simulink subsystem "Voice"  (R2023b)
settings: Solver=VariableStepAuto  StartTime=0.0  StopTime=10.0  RelTol=1e-3
model mask{rng_seeds=0, sample_dim_f=0}
  mask prompts: rng_seeds "rng seeds"; sample_dim_f "sample dim"
settings Model: Creator=Edp  LastModifiedBy=giorg

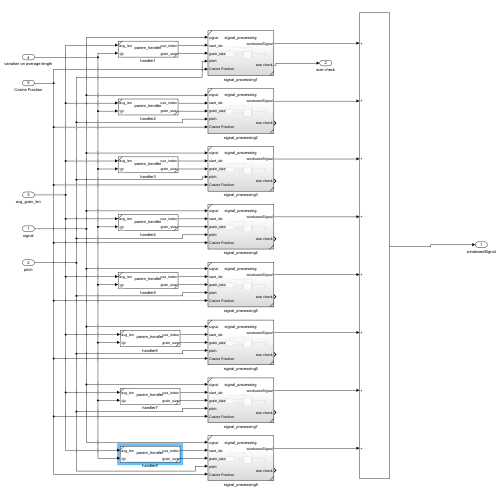
[thumbnail: Simulink's stored preview of the top-level diagram]
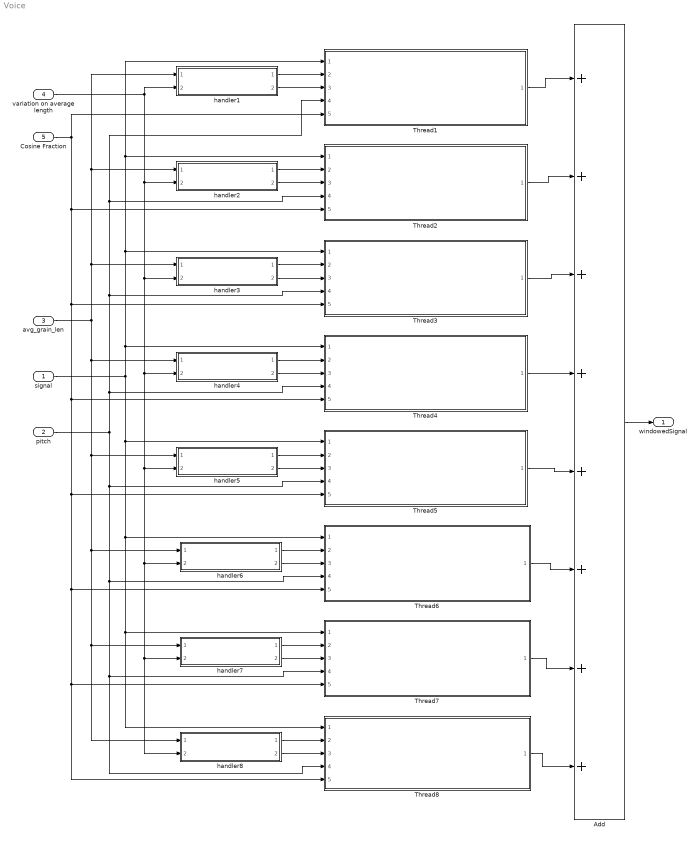
== system Voice ==
  signal : Inport
  pitch : Inport  Port=2
  avg_grain_len : Inport  Port=3
  variation on average length : Inport  Port=4
  Cosine Fraction : Inport  Port=5
  Add : Sum  Inputs=++++++++
  Thread{1..8} (8 alike) : Subsystem  ReferencedSubsystem=thread
  handler1 : Subsystem  ReferencedSubsystem=param_handler  rng_seed_f=rng_seeds(1)  sample_dim_f=sample_dim_f
  handler2 : Subsystem  ReferencedSubsystem=param_handler  rng_seed_f=rng_seeds(2)  sample_dim_f=sample_dim_f
  handler3 : Subsystem  ReferencedSubsystem=param_handler  rng_seed_f=rng_seeds(3)  sample_dim_f=sample_dim_f
  handler4 : Subsystem  ReferencedSubsystem=param_handler  rng_seed_f=rng_seeds(4)  sample_dim_f=sample_dim_f
  handler5 : Subsystem  ReferencedSubsystem=param_handler  rng_seed_f=rng_seeds(5)  sample_dim_f=sample_dim_f
  handler6 : Subsystem  ReferencedSubsystem=param_handler  rng_seed_f=rng_seeds(6)  sample_dim_f=sample_dim_f
  handler7 : Subsystem  ReferencedSubsystem=param_handler  rng_seed_f=rng_seeds(7)  sample_dim_f=sample_dim_f
  handler8 : Subsystem  ReferencedSubsystem=param_handler  rng_seed_f=rng_seeds(8)  sample_dim_f=sample_dim_f
  windowedSignal : Outport
  wires:
  handler1/2 -> Thread1/3
  handler1/1 -> Thread1/2
  Add/1 -> windowedSignal/1
  Thread1/1 -> Add/1
  Thread8/1 -> Add/8
  Thread7/1 -> Add/7
  Thread6/1 -> Add/6
  Thread5/1 -> Add/5
  Thread4/1 -> Add/4
  Thread3/1 -> Add/3
  Thread2/1 -> Add/2
  signal/1 -> Thread1/1, Thread2/1, Thread3/1, Thread4/1, Thread8/1, Thread7/1, Thread6/1, Thread5/1
  pitch/1 -> Thread5/4, Thread6/4, Thread7/4, Thread8/4, Thread1/4, Thread2/4, Thread3/4, Thread4/4
  handler2/1 -> Thread2/2
  handler2/2 -> Thread2/3
  handler3/1 -> Thread3/2
  handler3/2 -> Thread3/3
  handler4/1 -> Thread4/2
  handler4/2 -> Thread4/3
  handler5/1 -> Thread5/2
  handler5/2 -> Thread5/3
  handler6/1 -> Thread6/2
  handler6/2 -> Thread6/3
  handler7/1 -> Thread7/2
  handler7/2 -> Thread7/3
  handler8/1 -> Thread8/2
  handler8/2 -> Thread8/3
  avg_grain_len/1 -> handler3/1, handler2/1, handler1/1, handler4/1, handler5/1, handler6/1, handler8/1, handler7/1
  variation on average length/1 -> handler2/2, handler3/2, handler4/2, handler5/2, handler6/2, handler8/2, handler7/2, handler1/2
  Cosine Fraction/1 -> Thread1/5, Thread2/5, Thread8/5, Thread7/5, Thread6/5, Thread5/5, Thread4/5, Thread3/5
